simulink model "ES238A_HwAgArbn"  (R2013b)
settings: Solver=ode45  StartTime=0.0  StopTime=10  FixedStep=.002  RelTol=1e-3
values from neighbouring files (symbols this model uses):
  HwAgArbnHwAgMaxStall = DataDict.Calibration    [ES238A_HwAgArbn_DataDict.m]
  HWAGLIM_HWDEG_F32 = DataDict.Constant    [ES238A_HwAgArbn_DataDict.m]
undefined symbols (not defined in the file or in its folder): sigbuilder_block
libraries: simulink x4, NxtrLim x1
settings Model: Creator=rzqy0r  LastModifiedBy=nz3zln

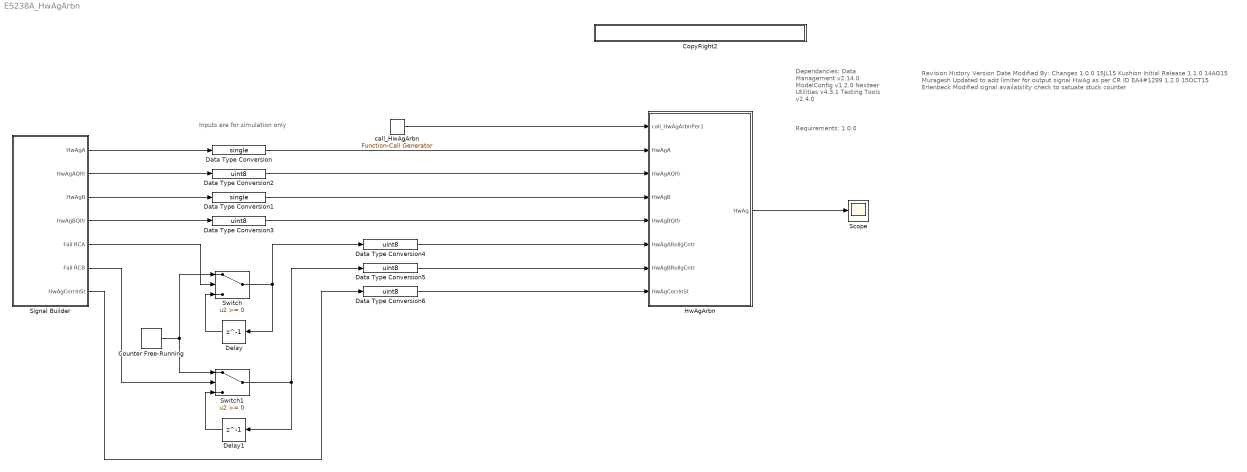
== system ES238A_HwAgArbn ==
  note: Inputs are for simulation only
  note: Revision History
      |
      | Version		Date 		Modified By: 		Changes
      | 1.0.0 		15JL15		Kushion			Initial Release
      | 1.1.0              14AG15        Muragesh             Updated to add limiter
      | 									       for output signal HwAg as per CR ID EA4#1299
      | 1.2.0               15OCT15     Erlenbeck             Modified signal availability check to satuate stuck counter
  note: Dependancies:
      |    Data Management v2.14.0
      |    ModelConfig v1.2.0
      |    Nexteer Utilities v4.3.1
      |    Testing Tools v2.4.0
  note: Requirements: 1.0.0
  CopyRight2 : Subsystem  Description=|  mask(Copyright Information){none=on}
      | Copyright info block.                                               
      |                                                                     
      | Place copyright information at the top of every subsystem in design.
      mask prompts: none "No parameters"
      mask help: Place copyright information at the top of every subsystem in design.
      mask Display:
      | NxtrConf = 'Nexteer Confidential';
      | 
      | sys = bdroot; %handle for the current model ("system")
      | first = get_param(sys,'Created');
      | first = first(end-3:end);  %year is last four digits
      | 
      | last = get_param(sys,'LastModifiedDate');
      | if isempty(last)
      |     last = datestr(now,'yyyy');
      | else
      |     last = last(end-3:end);
      | end
      | 
      | if strcmp(first,last)
      |     fprintf('%s -- Copyright %s Nexteer',NxtrConf,first)
      | else
      |     fprintf('%s -- %s%s- %s Nexteer',NxtrConf,char(169),first,last)
      | end
  Counter Free-Running : simulink/Sources/Counter Free-Running  NumBits=8  tsamp=0.004
  Data Type Conversion : DataTypeConversion  OutDataTypeStr=single
  Data Type Conversion1 : DataTypeConversion  OutDataTypeStr=single
  Data Type Conversion{2..6} (5 alike) : DataTypeConversion  OutDataTypeStr=uint8
  Delay : Delay  DelayLength=1  InitialCondition=0  SampleTime=0.004
  Delay1 : Delay  DelayLength=1  InitialCondition=0  SampleTime=0.004
  HwAgArbn : Subsystem
      settings: AttributesFormatString=%<Tag>
  Scope : Scope
      settings: YMin=0  YMax=850
  Signal Builder : Subsystem  Tag=STV Subsys  LoadFcn=sigbuilder_block('load',[234 -560.483 480.414 464.276 ]);  StartFcn=sigbuilder_block('start');  StopFcn=sigbuilder_block('stop');  ClipboardFcn=sigbuilder_block('clipboard');  mask(Sigbuilder block){}
      mask help: Simulink:masks:SigbuilderBlock_MD
      mask init:
      | if ~strcmp(get_param(bdroot(gcbh),'SimulationStatus'),'stopped') tuvar = sigbuilder_block('maskInit'); end
      settings: CopyFcn=sigbuilder_block('copy');  DeleteFcn=sigbuilder_block('delete');  ModelCloseFcn=sigbuilder_block('modelClose');  PreSaveFcn=sigbuilder_block('preSave');  PauseFcn=sigbuilder_block('pause');  ContinueFcn=sigbuilder_block('continue');  NameChangeFcn=sigbuilder_block('namechange');  OpenFcn=sigbuilder_block('open',[38.25 48.75 480.75 464.25 ]);  CloseFcn=sigbuilder_block('close');
      mask Display: plot(0, 0, 100, 100,[2, 2, 32, 32, 2], [68, 8, 8, 68, 68],[32, 2], [38, 38], [32, 19, 2],[53, 60, 44], [32, 17, 17, 2],[16, 16, 31, 31]);txt = getActiveGroup(gcbh);text(2, 100, txt,'verticalAlignment', 'top');
  Switch : Switch
  Switch1 : Switch
  call_HwAgArbn : simulink/Ports & Subsystems/Function-Call Generator  sample_time=.004  numberOfIterations=1
  wires:
  call_HwAgArbn/1 -> HwAgArbn/1(call_HwAgArbnPer1)
  Signal Builder/5(Fail RCA) -> Switch/2
  Delay/1 -> Switch/3
  Switch/1 -> Delay/1, Data Type Conversion4/1
  Counter Free-Running/1 -> Switch/1, Switch1/1
  Signal Builder/6(Fail RCB) -> Switch1/2
  Delay1/1 -> Switch1/3
  Switch1/1 -> Data Type Conversion5/1, Delay1/1
  Signal Builder/1(HwAgA) -> Data Type Conversion/1
  Signal Builder/2(HwAgAQlfr) -> Data Type Conversion2/1
  Signal Builder/3(HwAgB) -> Data Type Conversion1/1
  Signal Builder/4(HwAgBQlfr) -> Data Type Conversion3/1
  Data Type Conversion1/1 -> HwAgArbn/4(HwAgB)
  Data Type Conversion2/1 -> HwAgArbn/3(HwAgAQlfr)
  Data Type Conversion3/1 -> HwAgArbn/5(HwAgBQlfr)
  Data Type Conversion4/1 -> HwAgArbn/6(HwAgARollgCntr)
  Data Type Conversion5/1 -> HwAgArbn/7(HwAgBRollgCntr)
  Data Type Conversion/1 -> HwAgArbn/2(HwAgA)
  Signal Builder/7(HwAgCorrlnSt) -> Data Type Conversion6/1
  Data Type Conversion6/1 -> HwAgArbn/8(HwAgCorrlnSt)
  HwAgArbn/1(HwAg) -> Scope/1

== system ES238A_HwAgArbn/CopyRight2 ==

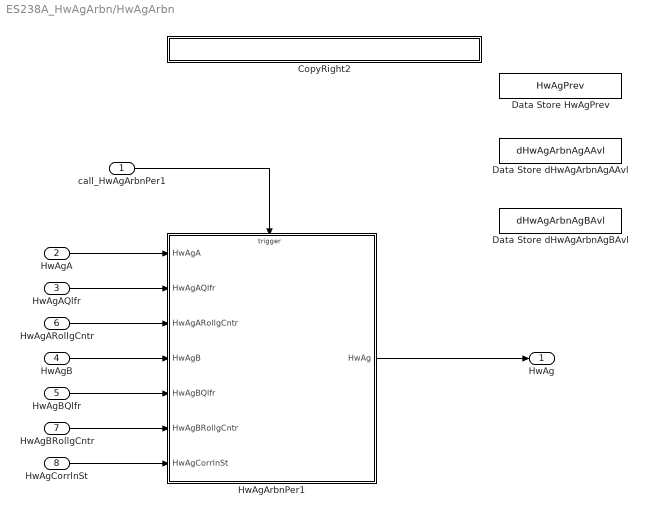
== system ES238A_HwAgArbn/HwAgArbn ==
  call_HwAgArbnPer1 : Inport
  HwAgA : Inport  Port=2  OutDataTypeStr=single
  HwAgAQlfr : Inport  Port=3
  HwAgB : Inport  Port=4  OutDataTypeStr=single
  HwAgBQlfr : Inport  Port=5
  HwAgARollgCntr : Inport  Port=6
  HwAgBRollgCntr : Inport  Port=7
  HwAgCorrlnSt : Inport  Port=8
  CopyRight2 : Subsystem  Description=|  mask(Copyright Information){none=on}
      | Copyright info block.                                               
      |                                                                     
      | Place copyright information at the top of every subsystem in design.
      mask prompts: none "No parameters"
      mask help: Place copyright information at the top of every subsystem in design.
      mask Display:
      | NxtrConf = 'Nexteer Confidential';
      | 
      | sys = bdroot; %handle for the current model ("system")
      | first = get_param(sys,'Created');
      | first = first(end-3:end);  %year is last four digits
      | 
      | last = get_param(sys,'LastModifiedDate');
      | if isempty(last)
      |     last = datestr(now,'yyyy');
      | else
      |     last = last(end-3:end);
      | end
      | 
      | if strcmp(first,last)
      |     fprintf('%s -- Copyright %s Nexteer',NxtrConf,first)
      | else
      |     fprintf('%s -- %s%s- %s Nexteer',NxtrConf,char(169),first,last)
      | end
  Data Store HwAgPrev : DataStoreMemory  DataStoreName=HwAgPrev
  Data Store dHwAgArbnAgAAvl : DataStoreMemory  DataStoreName=dHwAgArbnAgAAvl
  Data Store dHwAgArbnAgBAvl : DataStoreMemory  DataStoreName=dHwAgArbnAgBAvl
  HwAgArbnPer1 : Subsystem  Tag=0.002  TreatAsAtomicUnit=on
  HwAg : Outport
  wires:
  call_HwAgArbnPer1/1 -> HwAgArbnPer1/Trigger
  HwAgAQlfr/1 -> HwAgArbnPer1/2(HwAgAQlfr)
  HwAgARollgCntr/1 -> HwAgArbnPer1/3(HwAgARollgCntr)
  HwAgBQlfr/1 -> HwAgArbnPer1/5(HwAgBQlfr)
  HwAgBRollgCntr/1 -> HwAgArbnPer1/6(HwAgBRollgCntr)
  HwAgArbnPer1/1(HwAg) -> HwAg/1
  HwAgA/1 -> HwAgArbnPer1/1(HwAgA)
  HwAgB/1 -> HwAgArbnPer1/4(HwAgB)
  HwAgCorrlnSt/1 -> HwAgArbnPer1/7(HwAgCorrlnSt)

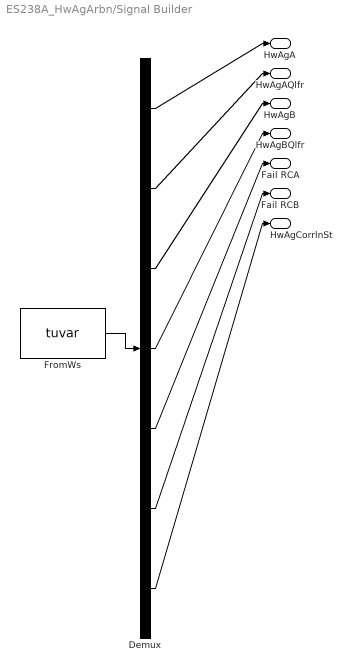
== system ES238A_HwAgArbn/Signal Builder ==
  Demux : Demux  Tag=STV Demux  Outputs=7
  FromWs : FromWorkspace  Tag=STV FromWs  VariableName=tuvar  SampleTime=0
      SigBuilderData=|
      | common.afterFinalStr = 'Extrapolate'
      | common.sampleTime = 0
      | dataSet(1).timeRange = [0 10]
      | dataSet(1).name = 'Normal Op'
      | dataSet(2).timeRange = [0 10]
      | dataSet(2).name = 'Correlation Failure'
      | dataSet(3).timeRange = [0 10]
      | dataSet(3).name = 'Qualifier A Failure Hold Last Value with Recovery'
      | dataSet(4).timeRange = [0 10]
      | dataSet(4).name = 'Short Qualifier A Failure - Confirm immediate Status but no indpt reduction'
      | dataSet(5).timeRange = [0 10]
      | dataSet(5).name = 'Qualifier A and B Failure with recovery'
      | sbobj.Groups(1).Name = 'Normal Op'
      | sbobj.Groups(1).Signals(1).Name = 'HwAgA'
      | sbobj.Groups(1).Signals(1).XData = [0 1 2 3 4 5 6 7 8 9 10]
      | sbobj.Groups(1).Signals(1).YData = [0 900 -900 900 -900 900 -222 180 0 0 0]
      | sbobj.Groups(1).Signals(2).Name = 'HwAgAQlfr'
      | sbobj.Groups(1).Signals(2).XData = [0 0.8 0.8 6 10]
      | sbobj.Groups(1).Signals(2).YData = [0 0 1 1 1]
      | sbobj.Groups(1).Signals(3).Name = 'HwAgB'
      | sbobj.Groups(1).Signals(3).XData = [0 1 2 3 4 5 6 7 8 9 10]
      | sbobj.Groups(1).Signals(3).YData = [0 900 -900 900 -900 900 -222 180 0 0 0]
      | sbobj.Groups(1).Signals(4).Name = 'HwAgBQlfr'
      | sbobj.Groups(1).Signals(4).XData = [0 1 1 2 10]
      | sbobj.Groups(1).Signals(4).YData = [0 0 1 1 1]
      | sbobj.Groups(1).Signals(5).Name = 'Fail RCA'
      | sbobj.Groups(1).Signals(5).XData = [0 4 6 10]
      | sbobj.Groups(1).Signals(5).YData = [1 1 1 1]
      | sbobj.Groups(1).Signals(6).Name = 'Fail RCB'
      | sbobj.Groups(1).Signals(6).XData = [0 4 6 10]
      | sbobj.Groups(1).Signals(6).YData = [1 1 1 1]
      | sbobj.Groups(1).Signals(7).Name = 'HwAgCorrlnSt'
      | sbobj.Groups(1).Signals(7).XData = [0 0.8 4 6 10]
      | sbobj.Groups(1).Signals(7).YData = [3 3 3 3 3]
      | sbobj.Groups(2).Name = 'Correlation Failure'
      | sbobj.Groups(2).Signals(1).Name = 'HwAgA'
      | sbobj.Groups(2).Signals(1).XData = [0 1 2 3 4 5 6 7 8 9 10]
      | sbobj.Groups(2).Signals(1).YData = [0 900 -900 900 -900 900 -222 180 0 0 0]
      | sbobj.Groups(2).Signals(2).Name = 'HwAgAQlfr'
      | sbobj.Groups(2).Signals(2).XData = [0 0.8 0.8 6 10]
      | sbobj.Groups(2).Signals(2).YData = [0 0 1 1 1]
      | sbobj.Groups(2).Signals(3).Name = 'HwAgB'
      | sbobj.Groups(2).Signals(3).XData = [0 1 2 3 4 5 6 7 8 9 10]
      | sbobj.Groups(2).Signals(3).YData = [0 900 -900 900 -900 900 -222 -264.9 0 0 0]
      | sbobj.Groups(2).Signals(4).Name = 'HwAgBQlfr'
      | sbobj.Groups(2).Signals(4).XData = [0 1 1 2 10]
      | sbobj.Groups(2).Signals(4).YData = [0 0 1 1 1]
      | sbobj.Groups(2).Signals(5).Name = 'Fail RCA'
      | sbobj.Groups(2).Signals(5).XData = [0 4 6 10]
      | sbobj.Groups(2).Signals(5).YData = [1 1 1 1]
      | sbobj.Groups(2).Signals(6).Name = 'Fail RCB'
      | sbobj.Groups(2).Signals(6).XData = [0 4 6 10]
      | sbobj.Groups(2).Signals(6).YData = [1 1 1 1]
      | sbobj.Groups(2).Signals(7).Name = 'HwAgCorrlnSt'
      | sbobj.Groups(2).Signals(7).XData = [0 0.8 4 6 10]
      | sbobj.Groups(2).Signals(7).YData = [3 3 3 3 3]
      | sbobj.Groups(3).Name = 'Qualifier A Failure Hold Last Value with Recovery'
      | sbobj.Groups(3).Signals(1).Name = 'HwAgA'
      | sbobj.Groups(3).Signals(1).XData = [0 1 2 3 4 5 6 7 8 9 10]
      | sbobj.Groups(3).Signals(1).YData = [0 900 -900 900 -900 900 -222 180 0 0 0]
      | sbobj.Groups(3).Signals(2).Name = 'HwAgAQlfr'
      | sbobj.Groups(3).Signals(2).XData = [0 0.8 0.8 6 10]
      | sbobj.Groups(3).Signals(2).YData = [0 0 1 1 1]
      | sbobj.Groups(3).Signals(3).Name = 'HwAgB'
      | sbobj.Groups(3).Signals(3).XData = [0 1 2 3 4 5 5 6 7 8 9 10]
      | sbobj.Groups(3).Signals(3).YData = [0 900 -900 -900 -900 -900 900 -222 180 0 0 0]
      | sbobj.Groups(3).Signals(4).Name = 'HwAgBQlfr'
      | sbobj.Groups(3).Signals(4).XData = [0 1 1 2 2 3 4 5 5 10]
      | sbobj.Groups(3).Signals(4).YData = [0 0 1 1 2 2 2 2 1 1]
      | sbobj.Groups(3).Signals(5).Name = 'Fail RCA'
      | sbobj.Groups(3).Signals(5).XData = [0 4 6 10]
      | sbobj.Groups(3).Signals(5).YData = [1 1 1 1]
      | sbobj.Groups(3).Signals(6).Name = 'Fail RCB'
      | sbobj.Groups(3).Signals(6).XData = [0 4 6 10]
      | sbobj.Groups(3).Signals(6).YData = [1 1 1 1]
      | sbobj.Groups(3).Signals(7).Name = 'HwAgCorrlnSt'
      | sbobj.Groups(3).Signals(7).XData = [0 0.8 4 6 10]
      | sbobj.Groups(3).Signals(7).YData = [3 3 3 3 3]
      | sbobj.Groups(4).Name = 'Short Qualifier A Failure - Confirm immediate Status but no indpt reduction'
      | sbobj.Groups(4).Signals(1).Name = 'HwAgA'
      | sbobj.Groups(4).Signals(1).XData = [0 1 2 3 4 5 6 7 8 9 10]
      | sbobj.Groups(4).Signals(1).YData = [0 900 -900 900 -900 900 -222 180 0 0 0]
      | sbobj.Groups(4).Signals(2).Name = 'HwAgAQlfr'
      | sbobj.Groups(4).Signals(2).XData = [0 0.8 0.8 6 10]
      | sbobj.Groups(4).Signals(2).YData = [0 0 1 1 1]
      | sbobj.Groups(4).Signals(3).Name = 'HwAgB'
      | sbobj.Groups(4).Signals(3).XData = [0 1 2 3 4 5 6 7 8 9 10]
      | sbobj.Groups(4).Signals(3).YData = [0 900 -900 900 -900 900 -222 180 0 0 0]
      | sbobj.Groups(4).Signals(4).Name = 'HwAgBQlfr'
      | sbobj.Groups(4).Signals(4).XData = [0 1 1 2 2 2.05 2.05 4 5 10]
      | sbobj.Groups(4).Signals(4).YData = [0 0 1 1 2 2 1 1 1 1]
      | sbobj.Groups(4).Signals(5).Name = 'Fail RCA'
      | sbobj.Groups(4).Signals(5).XData = [0 4 6 10]
      | sbobj.Groups(4).Signals(5).YData = [1 1 1 1]
      | sbobj.Groups(4).Signals(6).Name = 'Fail RCB'
      | sbobj.Groups(4).Signals(6).XData = [0 4 6 10]
      | sbobj.Groups(4).Signals(6).YData = [1 1 1 1]
      | sbobj.Groups(4).Signals(7).Name = 'HwAgCorrlnSt'
      | sbobj.Groups(4).Signals(7).XData = [0 0.8 4 6 10]
      | sbobj.Groups(4).Signals(7).YData = [3 3 3 3 3]
      | sbobj.Groups(5).Name = 'Qualifier A and B Failure with recovery'
      | sbobj.Groups(5).Signals(1).Name = 'HwAgA'
      | sbobj.Groups(5).Signals(1).XData = [0 1 2 3 4 5 6 6 7 8 9 10]
      | sbobj.Groups(5).Signals(1).YData = [0 900 -900 900 -900 -900 -900 -222 180 0 0 0]
      | sbobj.Groups(5).Signals(2).Name = 'HwAgAQlfr'
      | sbobj.Groups(5).Signals(2).XData = [0 0.8 0.8 4 4 6 6 10]
      | sbobj.Groups(5).Signals(2).YData = [0 0 1 1 2 2 1 1]
      | sbobj.Groups(5).Signals(3).Name = 'HwAgB'
      | sbobj.Groups(5).Signals(3).XData = [0 1 2 3 4 5 5 6 7 8 9 10]
      | sbobj.Groups(5).Signals(3).YData = [0 900 -900 -900 -900 -900 900 -222 180 0 0 0]
      | sbobj.Groups(5).Signals(4).Name = 'HwAgBQlfr'
      | sbobj.Groups(5).Signals(4).XData = [0 1 1 2 2 3 4 5 5 10]
      | sbobj.Groups(5).Signals(4).YData = [0 0 1 1 2 2 2 2 1 1]
      | sbobj.Groups(5).Signals(5).Name = 'Fail RCA'
      | sbobj.Groups(5).Signals(5).XData = [0 4 6 10]
      | sbobj.Groups(5).Signals(5).YData = [1 1 1 1]
      | sbobj.Groups(5).Signals(6).Name = 'Fail RCB'
      | sbobj.Groups(5).Signals(6).XData = [0 4 6 10]
      | sbobj.Groups(5).Signals(6).YData = [1 1 1 1]
      | sbobj.Groups(5).Signals(7).Name = 'HwAgCorrlnSt'
      | sbobj.Groups(5).Signals(7).XData = [0 0.8 4 6 10]
      | sbobj.Groups(5).Signals(7).YData = [3 3 3 3 3]
  HwAgA : Outport  Tag=STV Outport
  HwAgAQlfr : Outport  Tag=STV Outport  Port=2
  HwAgB : Outport  Tag=STV Outport  Port=3
  HwAgBQlfr : Outport  Tag=STV Outport  Port=4
  Fail RCA : Outport  Tag=STV Outport  Port=5
  Fail RCB : Outport  Tag=STV Outport  Port=6
  HwAgCorrlnSt : Outport  Tag=STV Outport  Port=7
  wires:
  FromWs/1 -> Demux/1
  Demux/1 -> HwAgA/1
  Demux/2 -> HwAgAQlfr/1
  Demux/3 -> HwAgB/1
  Demux/4 -> HwAgBQlfr/1
  Demux/5 -> Fail RCA/1
  Demux/6 -> Fail RCB/1
  Demux/7 -> HwAgCorrlnSt/1

== system ES238A_HwAgArbn/HwAgArbn/CopyRight2 ==

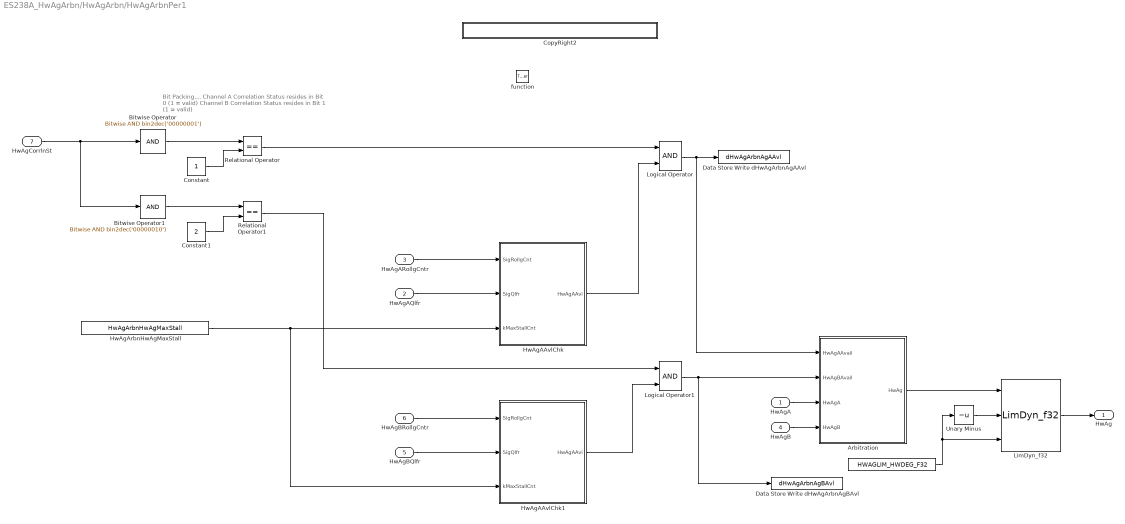
== system ES238A_HwAgArbn/HwAgArbn/HwAgArbnPer1 ==
  note: Bit Packing....
      | Channel A Correlation Status resides in Bit 0 (1 = valid)
      | Channel B Correlation Status resides in Bit 1 (1 = valid)
  HwAgA : Inport
  HwAgAQlfr : Inport  Port=2
  HwAgARollgCntr : Inport  Port=3
  HwAgB : Inport  Port=4
  HwAgBQlfr : Inport  Port=5
  HwAgBRollgCntr : Inport  Port=6
  HwAgCorrlnSt : Inport  Port=7
  function : TriggerPort  TriggerType=function-call
  " " : Constant  Value=HWAGLIM_HWDEG_F32
  Arbitration : Subsystem
  Bitwise Operator : simulink/Logic and Bit Operations/Bitwise Operator  RequirementInfo={'linktype_rmi_doors' '0000cf64 (/E-STEER Core/SubSystem Specifications/Electrical Actuator/Control Module/FDD Module Requirements/EA4/ES238A_HwAgArbn_Draft)' '#ES238A_35' 'true' 'REQ: ES238A_35' '' } %GIDa_bea3dfe8_bd46_4f20_9050_0a8791fa4549  logicop=AND  UseBitMask=on  BitMask=bin2dec('00000001')  BitMaskRealWorld=Stored Integer
  Bitwise Operator1 : simulink/Logic and Bit Operations/Bitwise Operator  RequirementInfo={'linktype_rmi_doors' '0000cf64 (/E-STEER Core/SubSystem Specifications/Electrical Actuator/Control Module/FDD Module Requirements/EA4/ES238A_HwAgArbn_Draft)' '#ES238A_69' 'true' 'REQ: ES238A_69' '' } %GIDa_3e7f2f7b_2dc6_46d9_9362_0e180cf441cb  logicop=AND  UseBitMask=on  BitMask=bin2dec('00000010')  BitMaskRealWorld=Stored Integer
  Constant : Constant  RequirementInfo={'linktype_rmi_doors' '0000cf64 (/E-STEER Core/SubSystem Specifications/Electrical Actuator/Control Module/FDD Module Requirements/EA4/ES238A_HwAgArbn_Draft)' '#ES238A_35' 'true' 'REQ: ES238A_35' '' } %GIDa_6ff7f489_96ba_46aa_b2f1_a64a9613b3ee  OutDataTypeStr=uint8
  Constant1 : Constant  RequirementInfo={'linktype_rmi_doors' '0000cf64 (/E-STEER Core/SubSystem Specifications/Electrical Actuator/Control Module/FDD Module Requirements/EA4/ES238A_HwAgArbn_Draft)' '#ES238A_69' 'true' 'REQ: ES238A_69' '' } %GIDa_f45f34c2_171a_44eb_a1df_4d6a4b1bffd2  Value=2  OutDataTypeStr=uint8
  CopyRight2 : Subsystem  Description=|  mask(Copyright Information){none=on}
      | Copyright info block.                                               
      |                                                                     
      | Place copyright information at the top of every subsystem in design.
      mask prompts: none "No parameters"
      mask help: Place copyright information at the top of every subsystem in design.
      mask Display:
      | NxtrConf = 'Nexteer Confidential';
      | 
      | sys = bdroot; %handle for the current model ("system")
      | first = get_param(sys,'Created');
      | first = first(end-3:end);  %year is last four digits
      | 
      | last = get_param(sys,'LastModifiedDate');
      | if isempty(last)
      |     last = datestr(now,'yyyy');
      | else
      |     last = last(end-3:end);
      | end
      | 
      | if strcmp(first,last)
      |     fprintf('%s -- Copyright %s Nexteer',NxtrConf,first)
      | else
      |     fprintf('%s -- %s%s- %s Nexteer',NxtrConf,char(169),first,last)
      | end
  Data Store Write dHwAgArbnAgAAvl : DataStoreWrite  DataStoreName=dHwAgArbnAgAAvl
  Data Store Write dHwAgArbnAgBAvl : DataStoreWrite  DataStoreName=dHwAgArbnAgBAvl
  HwAgAAvlChk : Subsystem  RequirementInfo={'linktype_rmi_doors' '0000cf64 (/E-STEER Core/SubSystem Specifications/Electrical Actuator/Control Module/FDD Module Requirements/EA4/ES238A_HwAgArbn)' '#ES238A_35' 'true' 'REQ: ES238A_35' '' } %GIDa_384c42cc_0ffd_45df_a9b6_fe81dd918992  TreatAsAtomicUnit=on
  HwAgAAvlChk1 : Subsystem  RequirementInfo={'linktype_rmi_doors' '0000cf64 (/E-STEER Core/SubSystem Specifications/Electrical Actuator/Control Module/FDD Module Requirements/EA4/ES238A_HwAgArbn)' '#ES238A_69' 'true' 'REQ: ES238A_69' '' } %GIDa_5614d209_ba0f_483c_adc9_19ace58ad118  TreatAsAtomicUnit=on
  HwAgArbnHwAgMaxStall : Constant  Value=HwAgArbnHwAgMaxStall
  LimDyn_f32 : NxtrLim/LimDyn_f32
  Logical Operator : Logic  RequirementInfo={'linktype_rmi_doors' '0000cf64 (/E-STEER Core/SubSystem Specifications/Electrical Actuator/Control Module/FDD Module Requirements/EA4/ES238A_HwAgArbn)' '#ES238A_35' 'true' 'REQ: ES238A_35' '' } %GIDa_74228a93_0199_43c7_a692_a5e35af96634  AllPortsSameDT=off  OutDataTypeStr=boolean
  Logical Operator1 : Logic  RequirementInfo={'linktype_rmi_doors' '0000cf64 (/E-STEER Core/SubSystem Specifications/Electrical Actuator/Control Module/FDD Module Requirements/EA4/ES238A_HwAgArbn)' '#ES238A_69' 'true' 'REQ: ES238A_69' '' } %GIDa_d6bc7edc_fcbb_45f5_84ba_9ea40a0cffc3  AllPortsSameDT=off  OutDataTypeStr=boolean
  Relational Operator : RelationalOperator  RequirementInfo={'linktype_rmi_doors' '0000cf64 (/E-STEER Core/SubSystem Specifications/Electrical Actuator/Control Module/FDD Module Requirements/EA4/ES238A_HwAgArbn_Draft)' '#ES238A_35' 'true' 'REQ: ES238A_35' '' } %GIDa_a4dfbfe0_37fd_46a5_994f_5fd593b15e89  Operator===  OutDataTypeStr=boolean
  Relational Operator1 : RelationalOperator  RequirementInfo={'linktype_rmi_doors' '0000cf64 (/E-STEER Core/SubSystem Specifications/Electrical Actuator/Control Module/FDD Module Requirements/EA4/ES238A_HwAgArbn_Draft)' '#ES238A_69' 'true' 'REQ: ES238A_69' '' } %GIDa_4509dfe5_9e57_4cc6_a8da_43c85336e675  Operator===  OutDataTypeStr=boolean
  Unary Minus : UnaryMinus
  HwAg : Outport
  wires:
  HwAgARollgCntr/1 -> HwAgAAvlChk/1(SigRollgCnt)
  HwAgAQlfr/1 -> HwAgAAvlChk/2(SigQlfr)
  HwAgArbnHwAgMaxStall/1 -> HwAgAAvlChk1/3(kMaxStallCnt), HwAgAAvlChk/3(kMaxStallCnt)
  HwAgB/1 -> Arbitration/4(HwAgB)
  HwAgA/1 -> Arbitration/3(HwAgA)
  HwAgCorrlnSt/1 -> Bitwise Operator1/1, Bitwise Operator/1
  Bitwise Operator/1 -> Relational Operator/1
  Constant/1 -> Relational Operator/2
  Constant1/1 -> Relational Operator1/2
  Bitwise Operator1/1 -> Relational Operator1/1
  Relational Operator1/1 -> Logical Operator1/1
  HwAgBRollgCntr/1 -> HwAgAAvlChk1/1(SigRollgCnt)
  HwAgBQlfr/1 -> HwAgAAvlChk1/2(SigQlfr)
  Relational Operator/1 -> Logical Operator/1
  Logical Operator/1 -> Arbitration/1(HwAgAAvail), Data Store Write dHwAgArbnAgAAvl/1
  HwAgAAvlChk/1(HwAgAAvl) -> Logical Operator/2
  HwAgAAvlChk1/1(HwAgAAvl) -> Logical Operator1/2
  Logical Operator1/1 -> Data Store Write dHwAgArbnAgBAvl/1, Arbitration/2(HwAgBAvail)
  " "/1 -> Unary Minus/1, LimDyn_f32/3
  Unary Minus/1 -> LimDyn_f32/2
  Arbitration/1(HwAg) -> LimDyn_f32/1
  LimDyn_f32/1 -> HwAg/1

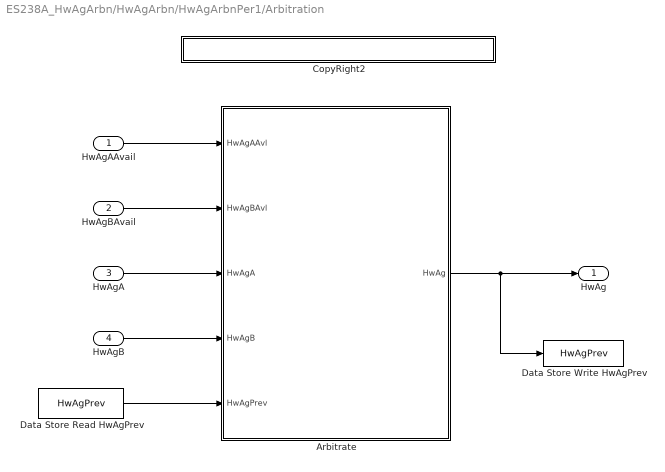
== system ES238A_HwAgArbn/HwAgArbn/HwAgArbnPer1/Arbitration ==
  HwAgAAvail : Inport
  HwAgBAvail : Inport  Port=2
  HwAgA : Inport  Port=3
  HwAgB : Inport  Port=4
  Arbitrate : Truth Table  RequirementInfo={'linktype_rmi_doors' '0000cf64 (/E-STEER Core/SubSystem Specifications/Electrical Actuator/Control Module/FDD Module Requirements/EA4/ES238A_HwAgArbn_Draft)' '#ES238A_108' 'true' 'REQ: ES238A_108' '' ; 'linktype_rmi_doors' '0000cf64 (/E-STEER Core/SubSystem Specifications/Electrical Actuator/Control Module/FDD Module Requirements/EA4/ES238A_HwAgArbn_Draft)' '#ES238A_84' 'true' 'REQ: ES238A_84' '' ; 'linktype_rmi_doors' '0000cf64 (/E-STEER Core/SubSystem Specifications/Electrical Actuator/Control Module/FDD Module Requirements/EA4/ES238A_HwAgArbn_Draft)' '#ES238A_100' 'true' 'REQ: ES238A_100' '' ; 'linktype_rmi_doors' '0000cf64 (/E-STEER Core/SubSystem Specifications/Electrical Actuator/Control Module/FDD Module Requirements/EA4/ES238A_HwAgArbn_Draft)' '#ES238A_106' 'true' 'REQ: ES238A_106' '' } %GIDa_fe6c1ad2_675b_4e65_b878_1274f9628793  TreatAsAtomicUnit=on
  CopyRight2 : Subsystem  Description=|  mask(Copyright Information){none=on}
      | Copyright info block.                                               
      |                                                                     
      | Place copyright information at the top of every subsystem in design.
      mask prompts: none "No parameters"
      mask help: Place copyright information at the top of every subsystem in design.
      mask Display:
      | NxtrConf = 'Nexteer Confidential';
      | 
      | sys = bdroot; %handle for the current model ("system")
      | first = get_param(sys,'Created');
      | first = first(end-3:end);  %year is last four digits
      | 
      | last = get_param(sys,'LastModifiedDate');
      | if isempty(last)
      |     last = datestr(now,'yyyy');
      | else
      |     last = last(end-3:end);
      | end
      | 
      | if strcmp(first,last)
      |     fprintf('%s -- Copyright %s Nexteer',NxtrConf,first)
      | else
      |     fprintf('%s -- %s%s- %s Nexteer',NxtrConf,char(169),first,last)
      | end
  Data Store Read HwAgPrev : DataStoreRead  DataStoreName=HwAgPrev
  Data Store Write HwAgPrev : DataStoreWrite  DataStoreName=HwAgPrev
  HwAg : Outport
  wires:
  HwAgBAvail/1 -> Arbitrate/2(HwAgBAvl)
  HwAgA/1 -> Arbitrate/3(HwAgA)
  HwAgAAvail/1 -> Arbitrate/1(HwAgAAvl)
  HwAgB/1 -> Arbitrate/4(HwAgB)
  Arbitrate/1(HwAg) -> Data Store Write HwAgPrev/1, HwAg/1
  Data Store Read HwAgPrev/1 -> Arbitrate/5(HwAgPrev)

== system ES238A_HwAgArbn/HwAgArbn/HwAgArbnPer1/CopyRight2 ==

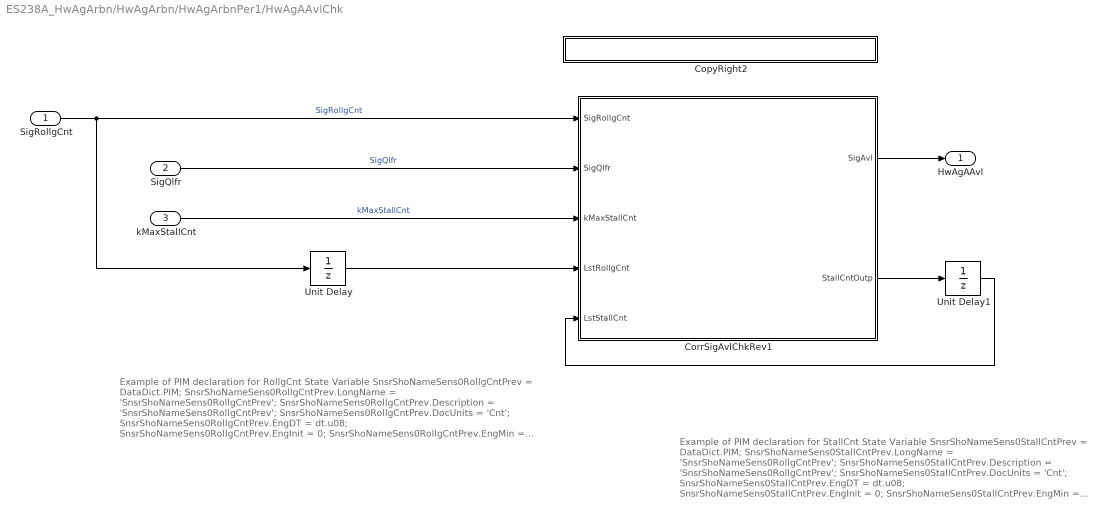
== system ES238A_HwAgArbn/HwAgArbn/HwAgArbnPer1/HwAgAAvlChk ==
  note: Example of PIM declaration for StallCnt State Variable
      |
      | SnsrShoNameSens0StallCntPrev = DataDict.PIM;
      | SnsrShoNameSens0StallCntPrev.LongName = 'SnsrShoNameSens0RollgCntPrev';
      | SnsrShoNameSens0StallCntPrev.Description = 'SnsrShoNameSens0RollgCntPrev';
      | SnsrShoNameSens0StallCntPrev.DocUnits = 'Cnt';
      | SnsrShoNameSens0StallCntPrev.EngDT = dt.u08;
      | SnsrShoNameSens0StallCntPrev.EngInit = 0;
      | SnsrShoNameSens0StallCntPrev.EngMin = 0;
      | SnsrShoNameSens0StallCntPrev.EngMax = 255;
      |
      |
      | *********  Need different state variable for each instance of this  subsystem ********
  note: Example of PIM declaration for RollgCnt State Variable
      |
      | SnsrShoNameSens0RollgCntPrev = DataDict.PIM;
      | SnsrShoNameSens0RollgCntPrev.LongName = 'SnsrShoNameSens0RollgCntPrev';
      | SnsrShoNameSens0RollgCntPrev.Description = 'SnsrShoNameSens0RollgCntPrev';
      | SnsrShoNameSens0RollgCntPrev.DocUnits = 'Cnt';
      | SnsrShoNameSens0RollgCntPrev.EngDT = dt.u08;
      | SnsrShoNameSens0RollgCntPrev.EngInit = 0;
      | SnsrShoNameSens0RollgCntPrev.EngMin = 0;
      | SnsrShoNameSens0RollgCntPrev.EngMax = 255;
      |
      |
      | *********  Need different state variable for each instance of this  subsystem ********
  SigRollgCnt : Inport  OutDataTypeStr=uint8
  SigQlfr : Inport  Port=2  OutDataTypeStr=uint8
  kMaxStallCnt : Inport  Port=3  OutDataTypeStr=uint8
  CopyRight2 : Subsystem  Description=|  mask(Copyright Information){none=on}
      | Copyright info block.                                               
      |                                                                     
      | Place copyright information at the top of every subsystem in design.
      mask prompts: none "No parameters"
      mask help: Place copyright information at the top of every subsystem in design.
      mask Display:
      | NxtrConf = 'Nexteer Confidential';
      | 
      | sys = bdroot; %handle for the current model ("system")
      | first = get_param(sys,'Created');
      | first = first(end-3:end);  %year is last four digits
      | 
      | last = get_param(sys,'LastModifiedDate');
      | if isempty(last)
      |     last = datestr(now,'yyyy');
      | else
      |     last = last(end-3:end);
      | end
      | 
      | if strcmp(first,last)
      |     fprintf('%s -- Copyright %s Nexteer',NxtrConf,first)
      | else
      |     fprintf('%s -- %s%s- %s Nexteer',NxtrConf,char(169),first,last)
      | end
  CorrSigAvlChkRev1 : Stateflow chart  TreatAsAtomicUnit=on
  Unit Delay : UnitDelay  SampleTime=-1  StateName=HwAgARollgCntrPrev  StateMustResolveToSignalObject=on
      settings: AttributesFormatString=|
      | State Variable:
      | %<StateName>
  Unit Delay1 : UnitDelay  SampleTime=-1  StateName=HwAgAStallCntrPrev  StateMustResolveToSignalObject=on
      settings: AttributesFormatString=|
      | State Variable:
      | %<StateName>
  HwAgAAvl : Outport
  wires:
  SigRollgCnt/1 -> CorrSigAvlChkRev1/1(SigRollgCnt), Unit Delay/1  "SigRollgCnt"
  SigQlfr/1 -> CorrSigAvlChkRev1/2(SigQlfr)  "SigQlfr"
  kMaxStallCnt/1 -> CorrSigAvlChkRev1/3(kMaxStallCnt)  "kMaxStallCnt"
  Unit Delay/1 -> CorrSigAvlChkRev1/4(LstRollgCnt)
  CorrSigAvlChkRev1/2(StallCntOutp) -> Unit Delay1/1
  Unit Delay1/1 -> CorrSigAvlChkRev1/5(LstStallCnt)
  CorrSigAvlChkRev1/1(SigAvl) -> HwAgAAvl/1

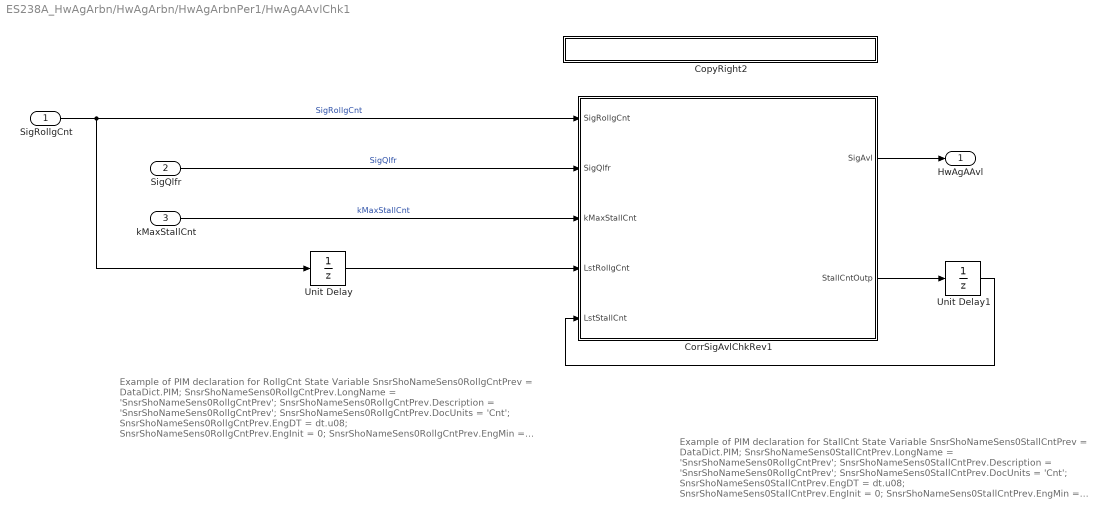
== system ES238A_HwAgArbn/HwAgArbn/HwAgArbnPer1/HwAgAAvlChk1 ==
  note: Example of PIM declaration for StallCnt State Variable
      |
      | SnsrShoNameSens0StallCntPrev = DataDict.PIM;
      | SnsrShoNameSens0StallCntPrev.LongName = 'SnsrShoNameSens0RollgCntPrev';
      | SnsrShoNameSens0StallCntPrev.Description = 'SnsrShoNameSens0RollgCntPrev';
      | SnsrShoNameSens0StallCntPrev.DocUnits = 'Cnt';
      | SnsrShoNameSens0StallCntPrev.EngDT = dt.u08;
      | SnsrShoNameSens0StallCntPrev.EngInit = 0;
      | SnsrShoNameSens0StallCntPrev.EngMin = 0;
      | SnsrShoNameSens0StallCntPrev.EngMax = 255;
      |
      |
      | *********  Need different state variable for each instance of this  subsystem ********
  note: Example of PIM declaration for RollgCnt State Variable
      |
      | SnsrShoNameSens0RollgCntPrev = DataDict.PIM;
      | SnsrShoNameSens0RollgCntPrev.LongName = 'SnsrShoNameSens0RollgCntPrev';
      | SnsrShoNameSens0RollgCntPrev.Description = 'SnsrShoNameSens0RollgCntPrev';
      | SnsrShoNameSens0RollgCntPrev.DocUnits = 'Cnt';
      | SnsrShoNameSens0RollgCntPrev.EngDT = dt.u08;
      | SnsrShoNameSens0RollgCntPrev.EngInit = 0;
      | SnsrShoNameSens0RollgCntPrev.EngMin = 0;
      | SnsrShoNameSens0RollgCntPrev.EngMax = 255;
      |
      |
      | *********  Need different state variable for each instance of this  subsystem ********
  SigRollgCnt : Inport  OutDataTypeStr=uint8
  SigQlfr : Inport  Port=2  OutDataTypeStr=uint8
  kMaxStallCnt : Inport  Port=3  OutDataTypeStr=uint8
  CopyRight2 : Subsystem  Description=|  mask(Copyright Information){none=on}
      | Copyright info block.                                               
      |                                                                     
      | Place copyright information at the top of every subsystem in design.
      mask prompts: none "No parameters"
      mask help: Place copyright information at the top of every subsystem in design.
      mask Display:
      | NxtrConf = 'Nexteer Confidential';
      | 
      | sys = bdroot; %handle for the current model ("system")
      | first = get_param(sys,'Created');
      | first = first(end-3:end);  %year is last four digits
      | 
      | last = get_param(sys,'LastModifiedDate');
      | if isempty(last)
      |     last = datestr(now,'yyyy');
      | else
      |     last = last(end-3:end);
      | end
      | 
      | if strcmp(first,last)
      |     fprintf('%s -- Copyright %s Nexteer',NxtrConf,first)
      | else
      |     fprintf('%s -- %s%s- %s Nexteer',NxtrConf,char(169),first,last)
      | end
  CorrSigAvlChkRev1 : Stateflow chart  TreatAsAtomicUnit=on
  Unit Delay : UnitDelay  SampleTime=-1  StateName=HwAgBRollgCntrPrev  StateMustResolveToSignalObject=on
      settings: AttributesFormatString=|
      | State Variable:
      | %<StateName>
  Unit Delay1 : UnitDelay  SampleTime=-1  StateName=HwAgBStallCntrPrev  StateMustResolveToSignalObject=on
      settings: AttributesFormatString=|
      | State Variable:
      | %<StateName>
  HwAgAAvl : Outport
  wires:
  SigRollgCnt/1 -> CorrSigAvlChkRev1/1(SigRollgCnt), Unit Delay/1  "SigRollgCnt"
  SigQlfr/1 -> CorrSigAvlChkRev1/2(SigQlfr)  "SigQlfr"
  kMaxStallCnt/1 -> CorrSigAvlChkRev1/3(kMaxStallCnt)  "kMaxStallCnt"
  Unit Delay/1 -> CorrSigAvlChkRev1/4(LstRollgCnt)
  CorrSigAvlChkRev1/2(StallCntOutp) -> Unit Delay1/1
  Unit Delay1/1 -> CorrSigAvlChkRev1/5(LstStallCnt)
  CorrSigAvlChkRev1/1(SigAvl) -> HwAgAAvl/1

== system ES238A_HwAgArbn/HwAgArbn/HwAgArbnPer1/Arbitration/CopyRight2 ==

== system ES238A_HwAgArbn/HwAgArbn/HwAgArbnPer1/HwAgAAvlChk/CopyRight2 ==

== system ES238A_HwAgArbn/HwAgArbn/HwAgArbnPer1/HwAgAAvlChk1/CopyRight2 ==

== stateflow chart ES238A_HwAgArbn/HwAgArbn/HwAgArbnPer1/HwAgAAvlChk1/CorrSigAvlChkRev1 ==
  note: SigAvl
      | False = 0
      | Pass = 1
  note: SigQlfr
      | 0 = No Result
      | 1 = Pass
      | 2 = Fail
  (default) -> (junction 2)
  (junction 2) -> (junction 4) [order 1] : [SigRollgCnt ==LstRollgCnt]
  (junction 4) -> (junction 7) [order 2] : {
      | StallCntOutp = LstStallCnt +1;
      | }
  (junction 2) -> (junction 3) [order 2]
  (junction 4) -> (junction 7) [order 1] : [LstStallCnt == 255]
      | {
      | StallCntOutp = 255;
      | }
  (junction 3) -> (junction 7) : {
      | StallCntOutp = 0;
      | }
  (junction 7) -> (junction 10)
  (junction 10) -> (junction 12) [order 1] : [StallCntOutp >=kMaxStallCnt]
  (junction 10) -> (junction 14) [order 2]
  (junction 12) -> (junction 17)
  (junction 14) -> (junction 17) [order 2]
  (junction 14) -> (junction 16) [order 1] : [SigQlfr<2]
  (junction 17) -> (junction 29) : {
      | SigAvl =0;
      | }
  (junction 16) -> (junction 29) : {
      | SigAvl = 1;
      | }
  data: SigRollgCnt input; SigQlfr input; kMaxStallCnt input; SigAvl output uint8; LstRollgCnt input uint8; LstStallCnt input uint8; StallCntOutp output uint8

== matlab function ES238A_HwAgArbn/HwAgArbn/HwAgArbnPer1/Arbitration/Arbitrate ==
  data: HwAg output single; HwAgAAvl input boolean; HwAgBAvl input boolean; HwAgA input single; HwAgB input single; HwAgPrev input single
function HwAg = fcn(HwAgAAvl, HwAgBAvl, HwAgA, HwAgB, HwAgPrev)

aVarTruthTableCondition_1 = false;
aVarTruthTableCondition_2 = false;


% HwAgA Available

aVarTruthTableCondition_1 = logical(HwAgAAvl);

% HwAgB Available

aVarTruthTableCondition_2 = logical(HwAgBAvl);

if (aVarTruthTableCondition_1 && aVarTruthTableCondition_2)
    aFcnTruthTableAction_1();
elseif (aVarTruthTableCondition_1 && ~aVarTruthTableCondition_2)
    aFcnTruthTableAction_2();
elseif (~aVarTruthTableCondition_1 && aVarTruthTableCondition_2)
    aFcnTruthTableAction_3();
else % Default
    aFcnTruthTableAction_4();
end

function aFcnTruthTableAction_1()

% Both signals available and with good correlation status

HwAg = (HwAgA + HwAgB)/2;

function aFcnTruthTableAction_2()

% Use Angle A

HwAg = HwAgA;

function aFcnTruthTableAction_3()

% Use Angle B

HwAg = HwAgB

function aFcnTruthTableAction_4()

% Use Previous Value

HwAg = HwAgPrev;

== stateflow chart ES238A_HwAgArbn/HwAgArbn/HwAgArbnPer1/HwAgAAvlChk/CorrSigAvlChkRev1 ==
  note: SigAvl
      | False = 0
      | Pass = 1
  note: SigQlfr
      | 0 = No Result
      | 1 = Pass
      | 2 = Fail
  (default) -> (junction 2)
  (junction 2) -> (junction 4) [order 1] : [SigRollgCnt ==LstRollgCnt]
  (junction 4) -> (junction 7) [order 2] : {
      | StallCntOutp = LstStallCnt +1;
      | }
  (junction 2) -> (junction 3) [order 2]
  (junction 4) -> (junction 7) [order 1] : [LstStallCnt == 255]
      | {
      | StallCntOutp = 255;
      | }
  (junction 3) -> (junction 7) : {
      | StallCntOutp = 0;
      | }
  (junction 7) -> (junction 10)
  (junction 10) -> (junction 12) [order 1] : [StallCntOutp >=kMaxStallCnt]
  (junction 10) -> (junction 14) [order 2]
  (junction 12) -> (junction 17)
  (junction 14) -> (junction 17) [order 2]
  (junction 14) -> (junction 16) [order 1] : [SigQlfr<2]
  (junction 17) -> (junction 29) : {
      | SigAvl =0;
      | }
  (junction 16) -> (junction 29) : {
      | SigAvl = 1;
      | }
  data: SigRollgCnt input; SigQlfr input; kMaxStallCnt input; SigAvl output uint8; LstRollgCnt input uint8; LstStallCnt input uint8; StallCntOutp output uint8
